simulink model "Delta_Sigma_ADC_Simplified_Blocks"  (R2012b)
settings: Solver=ode45  StartTime=0.0  StopTime=10.0  RelTol=1e-3
settings Model: Creator=ayush  LastModifiedBy=ayush
settings ConfigurationSet: Description=SimMechanics 2G

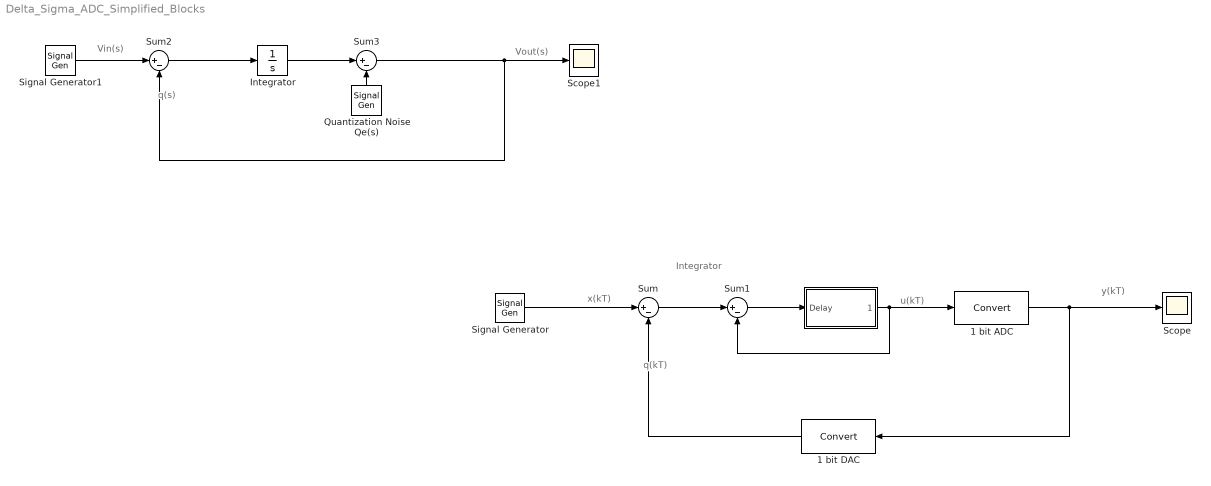
== system Delta_Sigma_ADC_Simplified_Blocks ==
  note: Vout(s)
  note: q(s)
  note: Vin(s)
  note: y(kT)
  note: u(kT)
  note: q(kT)
  note: x(kT)
  note: Integrator
  " " : Subsystem
  1 bit ADC : DataTypeConversion
  1 bit DAC : DataTypeConversion
  Integrator : Integrator
  Quantization Noise Qe(s) : SignalGenerator
  Scope : Scope
  Scope1 : Scope
  Signal Generator : SignalGenerator
  Signal Generator1 : SignalGenerator
  Sum{,1..3} (4 alike) : Sum  Inputs=|+-
  wires:
  Sum/1 -> Sum1/1
  " "/1(" ") -> Sum1/2, 1 bit ADC/1
  Sum1/1 -> " "/1("\t\t\t\t\t\t\tDelay")
  1 bit ADC/1 -> 1 bit DAC/1, Scope/1
  1 bit DAC/1 -> Sum/2
  Signal Generator/1 -> Sum/1
  Sum3/1 -> Scope1/1, Sum2/2
  Sum2/1 -> Integrator/1
  Integrator/1 -> Sum3/1
  Quantization Noise Qe(s)/1 -> Sum3/2
  Signal Generator1/1 -> Sum2/1

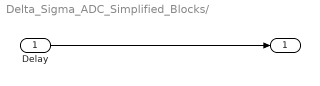
== system Delta_Sigma_ADC_Simplified_Blocks/  ==
  "\t\t\t\t\t\t\tDelay" : Inport
  " " : Outport
  wires:
  "\t\t\t\t\t\t\tDelay"/1 -> " "/1
